simulink model "PWM"  (R2020b)
settings: Solver=VariableStepAuto  StartTime=0.0  StopTime=10.0  RelTol=1e-3
libraries: simulink x1, powerlib_meascontrol x1
settings Model: Creator=MEDIA  LastModifiedBy=MEDIA

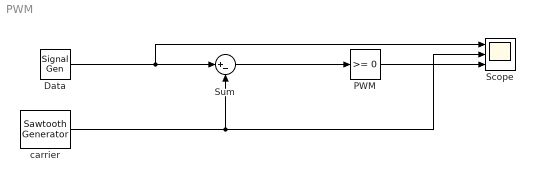
== system PWM ==
  Data : SignalGenerator  Amplitude=0.9  Units=rad/sec
  PWM : simulink/Logic and Bit Operations/Compare To Zero  relop=>=  OutDataTypeStr=boolean  ZeroCross=off
  Scope : Scope  NumInputPorts=3
  Sum : Sum  Inputs=|+-
  carrier : powerlib_meascontrol/Pulse & Signal Generators/Sawtooth Generator  Freq=1  Phase=0  Ts=0
  wires:
  Data/1 -> Scope/1, Sum/1
  Sum/1 -> PWM/1
  carrier/1 -> Scope/2, Sum/2
  PWM/1 -> Scope/3
